simulink subsystem "aero_fins"  (R2026a)
settings: Solver=VariableStepAuto
undefined symbols (not defined in the file or in its folder): fin_area, fin_aspectratio, fin_factor, fin_midchord_angle, fin_pos_x_cp, fin_pos_x_cp_mach2
settings Model: Creator=trist  LastModifiedBy=trist

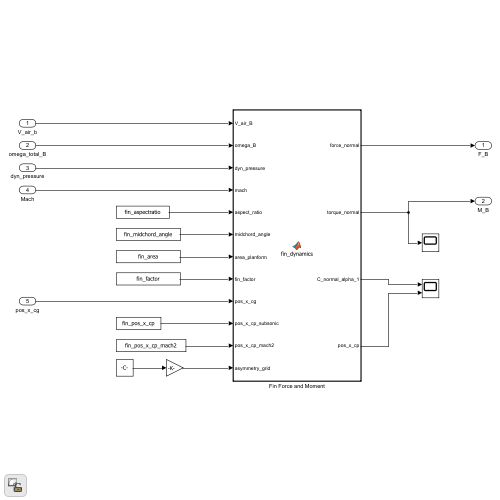
[thumbnail: Simulink's stored preview of the top-level diagram]
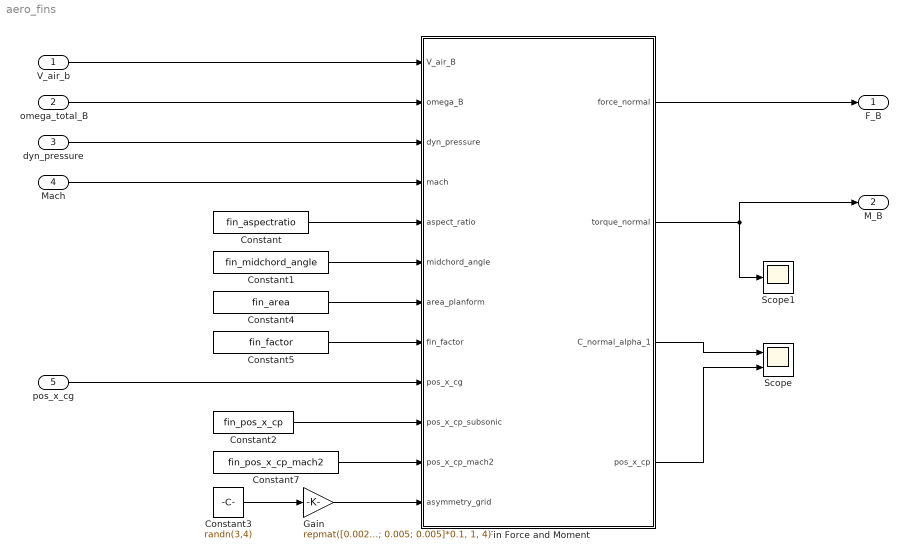
== system aero_fins ==
  V_air_b : Inport
  omega_total_B : Inport  Port=2
  "dyn_pressure " : Inport  Port=3
  "Mach " : Inport  Port=4
  pos_x_cg : Inport  Port=5
  Constant : Constant  Value=fin_aspectratio
  Constant1 : Constant  Value=fin_midchord_angle
  Constant2 : Constant  Value=fin_pos_x_cp
  Constant3 : Constant  Value=randn(3,4)  VectorParams1D=off
  Constant4 : Constant  Value=fin_area
  Constant5 : Constant  Value=fin_factor
  Constant7 : Constant  Value=fin_pos_x_cp_mach2
  Fin Force and Moment : MATLAB Function  TreatAsAtomicUnit=on
  Gain : Gain  Gain=repmat([0.002; 0.005; 0.005]*0.1, 1, 4)
  Scope : Scope  NumInputPorts=2
      settings: ActiveDisplayYMinimum=-5.7613098087759163  ActiveDisplayYMaximum=3.6048717258660559  DataLoggingVariableName=ScopeData16
  Scope1 : Scope
      settings: ActiveDisplayYMinimum=-1  ActiveDisplayYMaximum=1  DataLoggingVariableName=ScopeData17
  F_B : Outport
  M_B : Outport  Port=2  VectorParamsAs1DForOutWhenUnconnected=off
  wires:
  Constant/1 -> Fin Force and Moment/5(aspect_ratio)
  Constant1/1 -> Fin Force and Moment/6(midchord_angle)
  Constant4/1 -> Fin Force and Moment/7(area_planform)
  Constant5/1 -> Fin Force and Moment/8(fin_factor)
  Constant2/1 -> Fin Force and Moment/10(pos_x_cp_subsonic)
  pos_x_cg/1 -> Fin Force and Moment/9(pos_x_cg)
  Fin Force and Moment/3(C_normal_alpha_1) -> Scope/1
  Fin Force and Moment/1(force_normal) -> F_B/1
  "Mach "/1 -> Fin Force and Moment/4(mach)
  V_air_b/1 -> Fin Force and Moment/1(V_air_B)
  omega_total_B/1 -> Fin Force and Moment/2(omega_B)
  "dyn_pressure "/1 -> Fin Force and Moment/3(dyn_pressure)
  Fin Force and Moment/2(torque_normal) -> Scope1/1, M_B/1
  Fin Force and Moment/4(pos_x_cp) -> Scope/2
  Constant7/1 -> Fin Force and Moment/11(pos_x_cp_mach2)
  Constant3/1 -> Gain/1
  Gain/1 -> Fin Force and Moment/12(asymmetry_grid)

== matlab function aero_fins/Fin Force and Moment ==
  data: force_normal output; V_air_B input; omega_B input; dyn_pressure input; mach input; aspect_ratio input; midchord_angle input; area_planform input; fin_factor input; pos_x_cg input; torque_normal output; C_normal_alpha_1 output; pos_x_cp_subsonic input; pos_x_cp_mach2 input; pos_x_cp output; asymmetry_grid input
function [force_normal, torque_normal, C_normal_alpha_1, pos_x_cp] = fin_dynamics(V_air_B, omega_B, dyn_pressure, mach, aspect_ratio, midchord_angle, area_planform, fin_factor, pos_x_cg, pos_x_cp_subsonic, pos_x_cp_mach2, asymmetry_grid)
    %%% Calculate Theoretical Center of Pressure (Mach Dependent)
    subsonic = 0.6;
    supersonic = 1.6;
    
    if mach <= subsonic
        pos_x_cp = pos_x_cp_subsonic;
    elseif mach >= supersonic 
        pos_x_cp = pos_x_cp_mach2;
    else % Transonic Linear Interpolation
        ratio = (mach - supersonic) / (subsonic - supersonic); % Results in 0 to 1
        pos_x_cp = ratio * (pos_x_cp_subsonic - pos_x_cp_mach2) + pos_x_cp_mach2;
    end

    r_axial_ideal = (pos_x_cp - pos_x_cg) * [1; 0; 0]; 

    %%% Initialize Accumulators
    total_force = [0; 0; 0];
    total_torque = [0; 0; 0];
    sum_CN = 0;
    
    % Distribute the total fin factor across 4 fins
    % Intuitively this should be 4, however only 2 fins are 'active' at a
    % time (?). Also if the denominator is 4 we get instabilities. It's
    % probably worth further investigaion regardless.
    single_fin_scale = fin_factor / 2; 
    
    fin_angles = [0, pi/2, pi, 3*pi/2];
    
    %%% Loop Over Each Fin
    for i = 1:4
        theta = fin_angles(i);
        
        % Rotates about the X-axis by theta
        R_body_to_fin = [1, 0, 0;
                         0, cos(theta), sin(theta);
                         0, -sin(theta), cos(theta)];
        
        % Calculate Position (With Asymmetry)
        % Get the random manufacturing error for i-th fin
        fin_offset = asymmetry_grid(:, i); 
        pos_x_fin = r_axial_ideal + fin_offset;
        
        % Calculate Local Velocity at Fin Root
        V_local_body = V_air_B + cross(omega_B, pos_x_fin);
        
        % Rotate Velocity into Fin Frame
        V_fin = R_body_to_fin * V_local_body;
        
        % Calculate Incidence
        V_axial = V_fin(1);
        V_normal = V_fin(2);

        incidence = atan2(V_normal, V_axial);
        incidence_abs = abs(incidence);
        % Aerodynamic Coefficient
        CN_i = aerosurface_online(mach, incidence_abs, aspect_ratio, midchord_angle);
        sum_CN = sum_CN + CN_i; % For average calculation later
        
        % Calculate Force Magnitude
        F_mag = CN_i * single_fin_scale * dyn_pressure * area_planform * sin(incidence);
        
        % Force Direction (In Fin Frame)
        F_fin_frame = [0; F_mag; 0];
        
        % Rotate Force Back to Body Frame
        F_body_frame = R_body_to_fin' * F_fin_frame; % Transpose to inverse rotate
        
        % Calculate Torque
        T_body_frame = cross(F_body_frame, pos_x_fin);

        total_force = total_force + F_body_frame;
        total_torque = total_torque + T_body_frame;
    end
    
    %%% Final Outputs
    force_normal = total_force;
    torque_normal = total_torque;
    C_normal_alpha_1 = sum_CN / 4;
end
